simulink model "pwm_generator"  (R2015a)
settings: Solver=ode3  StartTime=0.0  StopTime=1  FixedStep=Ts  RelTol=1e-3
values from neighbouring files (symbols this model uses):
  Ts = 1/fs    (= 1e-05)    [VOC_param.m]    (also in VOC_param_paper.m = 5e-05; controller_parameters.m = 5e-05; power_control_param.m)
libraries: powerlib_meascontrol x2
settings Model: Creator=rblan  LastModifiedBy=rblan

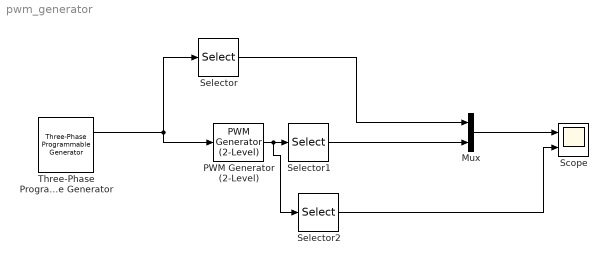
== system pwm_generator ==
  Mux : Mux  Inputs=2
  PWM Generator (2-Level) : powerlib_meascontrol/Pulse & Signal Generators/PWM Generator (2-Level)  ModulatorType=Three-phase bridge (6 pulses)  ModulatorMode=Unsynchronized  Fc=1000  Pc=90  nF=27  MinMax="[ -1  1 ]"  SamplingTechnique=Natural  ModulatingSignals=off  m=0.8  Freq=60  Phase=0  Ts=Ts  ShowCarrierOutport=off
  Scope : Scope  NumInputPorts=2
      settings: YMin=-5~-5  YMax=5~5
  Selector : Selector  InputPortWidth=3  Indices=[1]
  Selector1 : Selector  InputPortWidth=6  Indices=[1]
  Selector2 : Selector  InputPortWidth=6  Indices=[2]
  Three-Phase Programmable Generator : powerlib_meascontrol/Pulse & Signal Generators/Three-Phase Programmable Generator  Par_Vps=[1, 0, 50]  VariationEntity=None  VariationType=Ramp  VariationStep=-0.5  VariationRate=10  VariationMag=0.3  VariationFreq=2  Par_Timing_Variation="[0.2  1.2]"  SinglePhase=on  Yampli=[1 0.2 1.2 1.0]  Xtime=[0 0.1 0.15 0.2]  HarmonicGeneration=off  Par_HarmoA="[3  5  -25 0]"  Par_HarmoB="[5  10  35  2]"  Par_Timing_Harmo="[ 0.05  99]"  Ts=Ts
  wires:
  Three-Phase Programmable Generator/1 -> PWM Generator (2-Level)/1, Selector/1
  Mux/1 -> Scope/1
  Selector/1 -> Mux/1
  PWM Generator (2-Level)/1 -> Selector2/1, Selector1/1
  Selector1/1 -> Mux/2
  Selector2/1 -> Scope/2
